simulink model "Exercicio1"  (R2021a)
settings: Solver=VariableStepAuto  StartTime=0.0  StopTime=10.0  MaxStep=100  RelTol=1e-3
undefined symbols (not defined in the file or in its folder): A, B, C, D
settings Model: Creator=taffarel55  LastModifiedBy=taffarel55

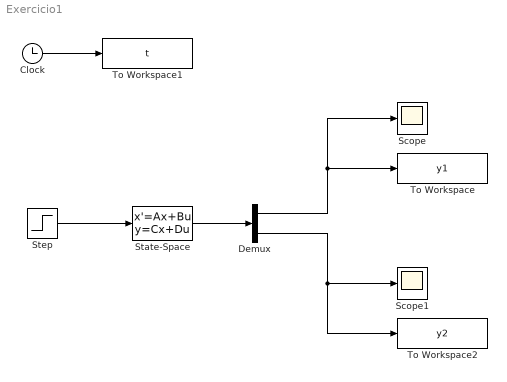
== system Exercicio1 ==
  Clock : Clock
  Demux : Demux  Outputs=2
  Scope : Scope
  Scope1 : Scope
  State-Space : StateSpace  A=A  B=B  C=C  D=D  InitialCondition=0
  Step : Step  SampleTime=0
  To Workspace : ToWorkspace  VariableName=y1  SaveFormat=Timeseries  SampleTime=-1
  To Workspace1 : ToWorkspace  VariableName=t  SaveFormat=Timeseries  SampleTime=-1
  To Workspace2 : ToWorkspace  VariableName=y2  SaveFormat=Timeseries  SampleTime=-1
  wires:
  Clock/1 -> To Workspace1/1
  Step/1 -> State-Space/1
  State-Space/1 -> Demux/1
  Demux/2 -> To Workspace2/1, Scope1/1
  Demux/1 -> Scope/1, To Workspace/1
